simulink model "EmbeddedPart3"  (R2018b)
settings: Solver=ode3  StartTime=0.0  StopTime=inf  RelTol=1e-3  EnableMultiTasking=on
libraries: legoev3lib x6
settings Model: FPTRunName=Active  ExtModeTrigDuration=2  Creator=Νίκος  LastModifiedBy=tom
settings SolverCC: PositivePriorityOrder=on
settings DataIOCC: LimitDataPoints=on  SaveFormat=Array
settings OptimizationCC: ExpressionDepthLimit=2147483647  LifeSpan=Inf  MaxStackSize=64
settings DebuggingCC: UnderspecifiedInitializationDetection=Classic  MergeDetectMultiDrivingBlocksExec=none  FcnCallInpInsideContextMsg=warning  AllowSymbolicDim=off  StateNameClashWarn=warning  SFUnexpectedBacktrackingDiag=warning  SFNoUnconditionalDefaultTransitionDiag=warning  SFExecutionAtInitializationDiag=none
settings HardwareCC: ProdBitPerPointer=32  ProdBitPerSizeT=32  ProdBitPerPtrDiffT=32  ProdLargestAtomicInteger=Long  ProdWordSize=32  ProdHWDeviceType=ARM Compatible->ARM 9  UseEmbeddedCoderFeatures=off  UseSimulinkCoderFeatures=off
settings ModelReferenceCC: PropagateSignalLabelsOutOfModel=off
settings SFSimCC: SimUseLocalCustomCode=off
settings RTWCC: SystemTargetFile=ert.tlc  HardwareBoard=LEGO MINDSTORMS EV3  TemplateMakefile=ert_default_tmf  GenerateReport=on  RTWVerbose=off  RTWUseLocalCustomCode=off  Toolchain=Sourcery G++ Lite v2009q3  BuildConfiguration=Faster Runs  LaunchReport=on
settings CodeAppCC: ForceParamTrailComments=on  OperatorAnnotations=on  StateflowObjectComments=on  MATLABSourceComments=on
settings ERTTargetCC: MultiwordLength=2048  ERTCustomFileBanners=off  SupportContinuousTime=on  SupportNonInlinedSFcns=on  RemoveResetFunc=off  SupportVariableSizeSignals=on  ModelStepFunctionPrototypeControlCompliant=off
settings ConfigComp: CovMetricSettings=dw  CovHtmlReporting=on  CovSaveCumulativeToWorkspaceVar=on  CovSaveSingleToWorkspaceVar=on  CovExternalEMLEnable=off  CovSFcnEnable=off

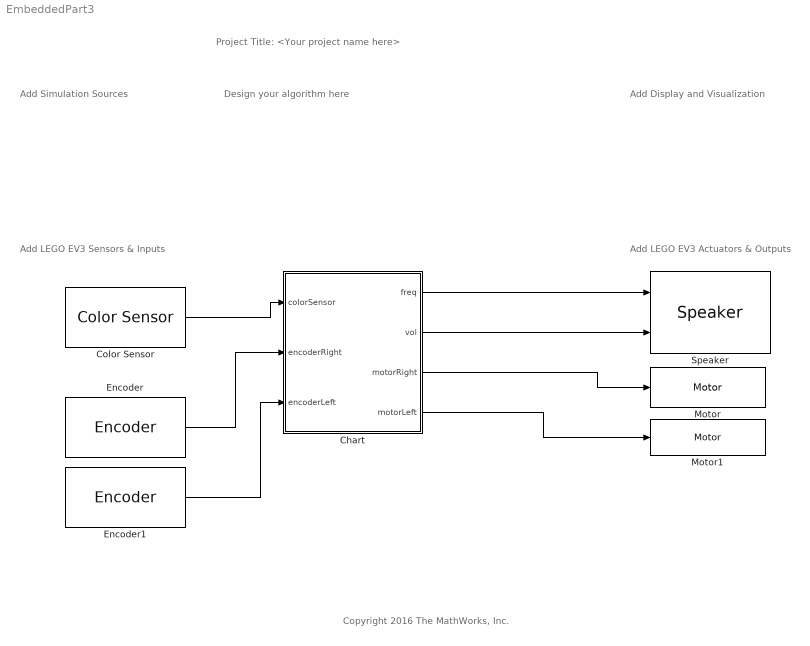
== system EmbeddedPart3 ==
  note: Project Title: <Your project name here>
  note: Copyright 2016 The MathWorks, Inc.
  note: Add LEGO EV3 Sensors & Inputs
  note: Add LEGO EV3 Actuators & Outputs
  note: Add Display and Visualization
  note: Design your algorithm here
  note: Add Simulation Sources
  Chart : Stateflow chart  TreatAsAtomicUnit=on
  Color Sensor : legoev3lib/Color Sensor  portNumber=3  mode=Color  sampleTime=0.1
      settings: SourceProductName=Simulink Support Package for LEGO MINDSTORMS EV3 Hardware  SourceProductBaseCode=LEGOEV3
  Encoder : legoev3lib/Encoder  portNumber=C  opMode=Reset by external signal  sampleTime=0.1
      settings: SourceProductName=Simulink Support Package for LEGO MINDSTORMS EV3 Hardware  SourceProductBaseCode=LEGOEV3
  Encoder1 : legoev3lib/Encoder  portNumber=B  opMode=Reset by external signal  sampleTime=0.1
      settings: SourceProductName=Simulink Support Package for LEGO MINDSTORMS EV3 Hardware  SourceProductBaseCode=LEGOEV3
  Motor : legoev3lib/Motor  sportNumber=C  sstopAction=Brake
  Motor1 : legoev3lib/Motor  sportNumber=B  sstopAction=Brake
  Speaker : legoev3lib/Speaker  sinputMode=Frequency and volume  sspeakerFreq=100  sspeakerVolume=50  sspeakerDuration=500
      settings: SourceProductName=Simulink Support Package for LEGO MINDSTORMS EV3 Hardware  SourceProductBaseCode=LEGOEV3
  wires:
  Chart/1(freq) -> Speaker/1
  Chart/2(vol) -> Speaker/2
  Chart/3(motorRight) -> Motor/1
  Chart/4(motorLeft) -> Motor1/1
  Color Sensor/1 -> Chart/1(colorSensor)
  Encoder/1 -> Chart/2(encoderRight)
  Encoder1/1 -> Chart/3(encoderLeft)

== stateflow chart EmbeddedPart3/Chart ==
  state BeepAndTurn
    entry:
    freq = 600;
    vol = 100;
    motorLeft = 100;
    motorRight = -100;
  state MoveForward
    entry:
    freq = 0;
    vol = 0;
    motorLeft = 100;
    motorRight = 100;
  state StopRobot
    entry:
    motorLeft = 0;
    motorRight = 0;
  state Beep
    entry:
    freq = 600;
    vol = 100;
  state BeepStop
    entry:
    freq = 0;
    vol = 0;
  state PauseRealQuick
    entry:
    motorLeft = 0;
    motorRight = 0;
  (default) -> BeepAndTurn
  PauseRealQuick -> MoveForward : after(0.2, sec)
  MoveForward -> StopRobot : [after(0.5, sec)]
  StopRobot -> Beep : [after(0.5, sec)]
  Beep -> BeepStop : [after(0.5, sec)]
  BeepAndTurn -> PauseRealQuick : [encoderLeft - encoderRight > 3 * 90]
  data: freq output; vol output; motorRight output; motorLeft output; colorSensor input; encoderRight input; encoderLeft input
